simulink model "sparse_learning_filter"  (R2021b)
settings: Solver=FixedStepDiscrete  StartTime=0.0  StopTime=10.0  FixedStep=0.5  RelTol=1e-3
libraries: wnnlib x24
settings Model: Creator=20214358  LastModifiedBy=20214358

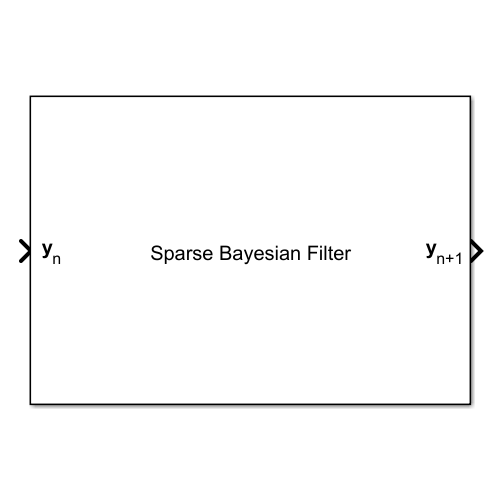
[thumbnail: Simulink's stored preview of the top-level diagram]
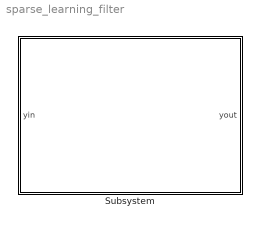
== system sparse_learning_filter ==
  Subsystem : Subsystem
      mask Display:
      | disp('Sparse Bayesian Filter','interpreter','tex');
      | port_label('input', 1,'{\bf y}_{n}','interpreter','tex');
      | port_label('output', 1,'{\bf y}_{n+1}','interpreter','tex');

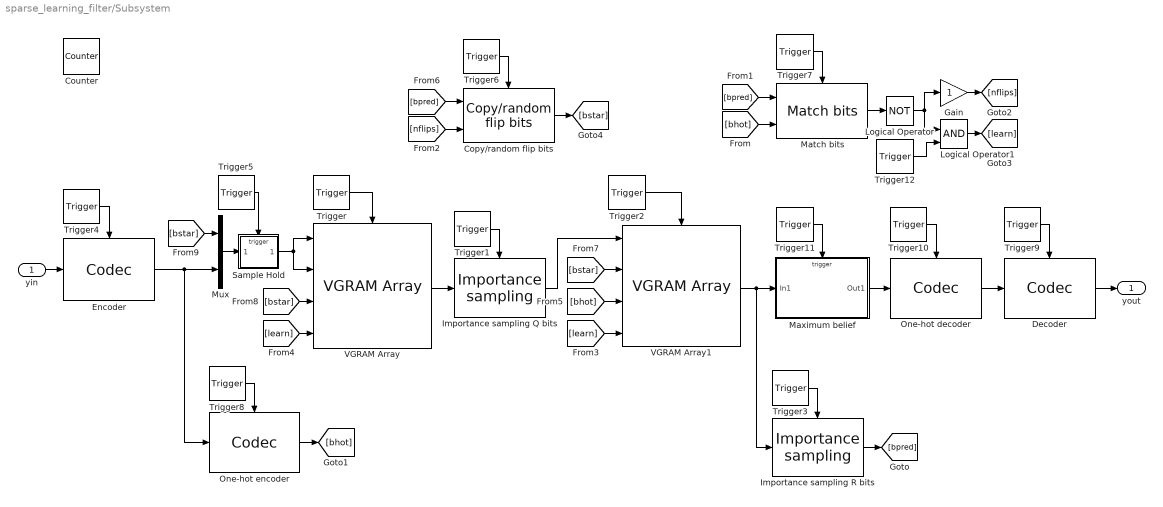
== system sparse_learning_filter/Subsystem ==
  yin : Inport
  Copy/random flip bits : wnnlib/Utilities/Copy//random flip bits
      settings: SourceProductName=Weightless Neural Networks Toolbox
  Counter : wnnlib/Sources/Counter  number_of_steps=9  sample_time=-1
      settings: SourceProductName=Weightless Neural Networks Toolbox
  Decoder : wnnlib/Utilities/Codec  codec_id=0  dense_vector_length=2  sparse_vector_length=2048  max_depth=16  learning_rate=0.0000001  min_splitting_volume=0.00001  min_bounds=[-10 -10]  max_bounds=[10 10]  sparse_vectors_file=C:\Users\20214358\MATLAB\Projects\wnnlib\wnndata\64k_sparse_vectors_seed_0.npz  debug_flag=off  codec_type=Decoder  number_of_sparse_vectors=65536
      settings: SourceProductName=Weightless Neural Networks Toolbox
  Encoder : wnnlib/Utilities/Codec  codec_id=0  dense_vector_length=2  sparse_vector_length=2048  max_depth=16  learning_rate=0.0000001  min_splitting_volume=0.00001  min_bounds=[-10 -10]  max_bounds=[10 10]  sparse_vectors_file=C:\Users\20214358\MATLAB\Projects\wnnlib\wnndata\64k_sparse_vectors_seed_0.npz  debug_flag=off  codec_type=Encoder  number_of_sparse_vectors=65536
      settings: SourceProductName=Weightless Neural Networks Toolbox
  Gain : Gain
  Importance sampling Q bits : wnnlib/Utilities/Importance sampling  nSamples=8
      settings: SourceProductName=Weightless Neural Networks Toolbox
  Importance sampling R bits : wnnlib/Utilities/Importance sampling  nSamples=8
      settings: SourceProductName=Weightless Neural Networks Toolbox
  Logical Operator : Logic  Operator=NOT  IconShape=distinctive  AllPortsSameDT=off  OutDataTypeStr=boolean
  Logical Operator1 : Logic  IconShape=distinctive  AllPortsSameDT=off  OutDataTypeStr=boolean
  Match bits : wnnlib/Utilities/Match bits  nMatchTolerance=1
      settings: SourceProductName=Weightless Neural Networks Toolbox
  Maximum belief : Subsystem  TreatAsAtomicUnit=on  mask{nSamples=8}
      mask prompts: nSamples "Number of samples"
      mask help: Build an unnormalized belief from a histogram collecting the frequencies among a finite number of discrete states. The belief is encoded as a sparse binary sequence with the same length as the number of discrete states. However, it comprises a small number of ones (samples) among several zeros such that the likelihood of a discrete space being assigned to one is proportional to its corresponding frequency in the histogram.
      mask init:
      | assert(nSamples > 0, 'Number of samples must be greater than zero.')
      mask Display:
      | disp('\ldots,0,1,0,\ldots','interpreter','tex');
      | port_label('input', 1,'{\bf h}','interpreter','tex')
      | port_label('output', 1,'{\bf b}','interpreter','tex')
      | port_label('trigger','\uparrow','interpreter','tex')
  Mux : Mux  Inputs=2
  One-hot decoder : wnnlib/Utilities/Codec  codec_id=0  dense_vector_length=2  sparse_vector_length=2048  max_depth=16  learning_rate=0.0000001  min_splitting_volume=0.00001  min_bounds=[-10 -10]  max_bounds=[10 10]  sparse_vectors_file=C:\Users\20214358\MATLAB\Projects\wnnlib\wnndata\64k_sparse_vectors_seed_0.npz  debug_flag=off  codec_type=OneHotDecoder  number_of_sparse_vectors=65536
      settings: SourceProductName=Weightless Neural Networks Toolbox
  One-hot encoder : wnnlib/Utilities/Codec  codec_id=0  dense_vector_length=2  sparse_vector_length=2048  max_depth=16  learning_rate=0.0000001  min_splitting_volume=0.00001  min_bounds=[-10 -10]  max_bounds=[10 10]  sparse_vectors_file=C:\Users\20214358\MATLAB\Projects\wnnlib\wnndata\64k_sparse_vectors_seed_0.npz  debug_flag=off  codec_type=OneHotEncoder  number_of_sparse_vectors=65536
      settings: SourceProductName=Weightless Neural Networks Toolbox
  Sample Hold : Subsystem  TreatAsAtomicUnit=on
      mask Display:
      | disp('S/H','interpreter','tex');
      | 
      | port_label('trigger','\uparrow','interpreter','tex');
  Trigger : wnnlib/Sources/Trigger  selected_steps=[2 8]
      settings: SourceProductName=Weightless Neural Networks Toolbox
  Trigger1 : wnnlib/Sources/Trigger  selected_steps=3
      settings: SourceProductName=Weightless Neural Networks Toolbox
  Trigger10 : wnnlib/Sources/Trigger  selected_steps=6
      settings: SourceProductName=Weightless Neural Networks Toolbox
  Trigger11 : wnnlib/Sources/Trigger  selected_steps=5
      settings: SourceProductName=Weightless Neural Networks Toolbox
  Trigger12 : wnnlib/Sources/Trigger  selected_steps=8
      settings: SourceProductName=Weightless Neural Networks Toolbox
  Trigger2 : wnnlib/Sources/Trigger  selected_steps=4|8
      settings: SourceProductName=Weightless Neural Networks Toolbox
  Trigger3 : wnnlib/Sources/Trigger  selected_steps=5
      settings: SourceProductName=Weightless Neural Networks Toolbox
  Trigger4 : wnnlib/Sources/Trigger  selected_steps=0
      settings: SourceProductName=Weightless Neural Networks Toolbox
  Trigger5 : wnnlib/Sources/Trigger  selected_steps=9
      settings: SourceProductName=Weightless Neural Networks Toolbox
  Trigger6 : wnnlib/Sources/Trigger  selected_steps=7
      settings: SourceProductName=Weightless Neural Networks Toolbox
  Trigger7 : wnnlib/Sources/Trigger  selected_steps=6
      settings: SourceProductName=Weightless Neural Networks Toolbox
  Trigger8 : wnnlib/Sources/Trigger  selected_steps=1
      settings: SourceProductName=Weightless Neural Networks Toolbox
  Trigger9 : wnnlib/Sources/Trigger  selected_steps=7
      settings: SourceProductName=Weightless Neural Networks Toolbox
  VGRAM Array : wnnlib/Models/VGRAM Array  array_id=0  min_mem_size=65535  max_mem_size=65536  min_dist=2  max_dist=8  pattern_length=16  output_dims=[4, 4]  debug_flag=on
      settings: SourceProductName=Weightless Neural Networks Toolbox
  VGRAM Array1 : wnnlib/Models/VGRAM Array  array_id=0  min_mem_size=65535  max_mem_size=65536  min_dist=2  max_dist=8  pattern_length=16  output_dims=[4, 4]  debug_flag=on
      settings: SourceProductName=Weightless Neural Networks Toolbox
  yout : Outport
  wires:
  Encoder/1 -> One-hot encoder/1, Mux/2
  Trigger1/1 -> Importance sampling Q bits/Trigger
  [learn] -> VGRAM Array1/4
  VGRAM Array1/1 -> Maximum belief/1(In1), Importance sampling R bits/1
  yin/1 -> Encoder/1
  Trigger2/1 -> VGRAM Array1/Trigger
  VGRAM Array/1 -> Importance sampling Q bits/1
  Importance sampling Q bits/1 -> VGRAM Array1/1
  Trigger4/1 -> Encoder/Trigger
  Trigger7/1 -> Match bits/Trigger
  Trigger6/1 -> Copy/random flip bits/Trigger
  Match bits/1 -> Logical Operator/1
  Trigger/1 -> VGRAM Array/Trigger
  [bhot] -> Match bits/2
  Trigger5/1 -> Sample Hold/Trigger
  Trigger3/1 -> Importance sampling R bits/Trigger
  [bpred] -> Match bits/1
  Logical Operator/1 -> Logical Operator1/1, Gain/1
  [nflips] -> Copy/random flip bits/2
  Gain/1 -> [nflips]
  Importance sampling R bits/1 -> [bpred]
  [bstar] -> VGRAM Array/3
  [learn] -> VGRAM Array/4
  Trigger8/1 -> One-hot encoder/Trigger
  One-hot encoder/1 -> [bhot]
  [bhot] -> VGRAM Array1/3
  [bpred] -> Copy/random flip bits/1
  Copy/random flip bits/1 -> [bstar]
  [bstar] -> VGRAM Array1/2
  Decoder/1 -> yout/1
  Trigger9/1 -> Decoder/Trigger
  Mux/1 -> Sample Hold/1(In1)
  Sample Hold/1(Out1) -> VGRAM Array/2, VGRAM Array/1
  [bstar] -> Mux/1
  One-hot decoder/1 -> Decoder/1
  Trigger10/1 -> One-hot decoder/Trigger
  Maximum belief/1(Out1) -> One-hot decoder/1
  Trigger11/1 -> Maximum belief/Trigger
  Logical Operator1/1 -> [learn]
  Trigger12/1 -> Logical Operator1/2

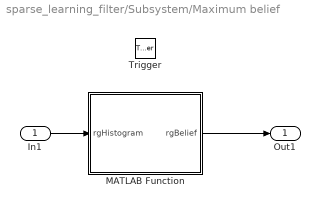
== system sparse_learning_filter/Subsystem/Maximum belief ==
  In1 : Inport
  Trigger : TriggerPort  VariantControl=(inherit)
  MATLAB Function : MATLAB Function  TreatAsAtomicUnit=on
  Out1 : Outport  OutDataTypeStr=uint8
  wires:
  MATLAB Function/1(rgBelief) -> Out1/1
  In1/1 -> MATLAB Function/1(rgHistogram)

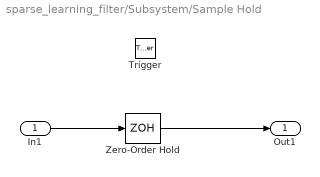
== system sparse_learning_filter/Subsystem/Sample Hold ==
  In1 : Inport
  Trigger : TriggerPort  VariantControl=(inherit)
  Zero-Order Hold : ZeroOrderHold  SampleTime=-1
  Out1 : Outport
  wires:
  In1/1 -> Zero-Order Hold/1
  Zero-Order Hold/1 -> Out1/1

== matlab function sparse_learning_filter/Subsystem/Maximum belief/MATLAB Function ==
  data: rgHistogram input; rgBelief output
function rgBelief = fcn(rgHistogram)


% Get the number of histogram dimensions
rgDims=size(rgHistogram);

% Initialize the unnormalized belief as all zeros
rgBelief = zeros(rgDims, 'uint8');

% Get the index of the maximum value
[~, idx] = max(rgBelief);

% Assign a value one to the selected discrete state
rgBelief(idx) = uint8(1);
